simulink model "untitle2d"  (R2022a)
settings: Solver=FixedStepAuto  StartTime=0.0  StopTime=50  FixedStep=0.1  RelTol=1e-3
undefined symbols (not defined in the file): c1, k1, m1
settings Model: Creator=sucho  LastModifiedBy=sucho

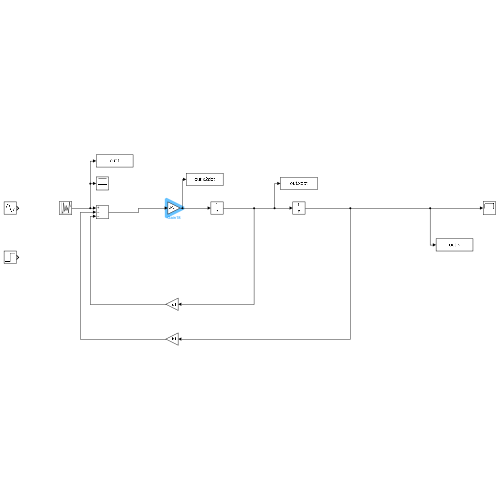
[thumbnail: Simulink's stored preview of the top-level diagram]
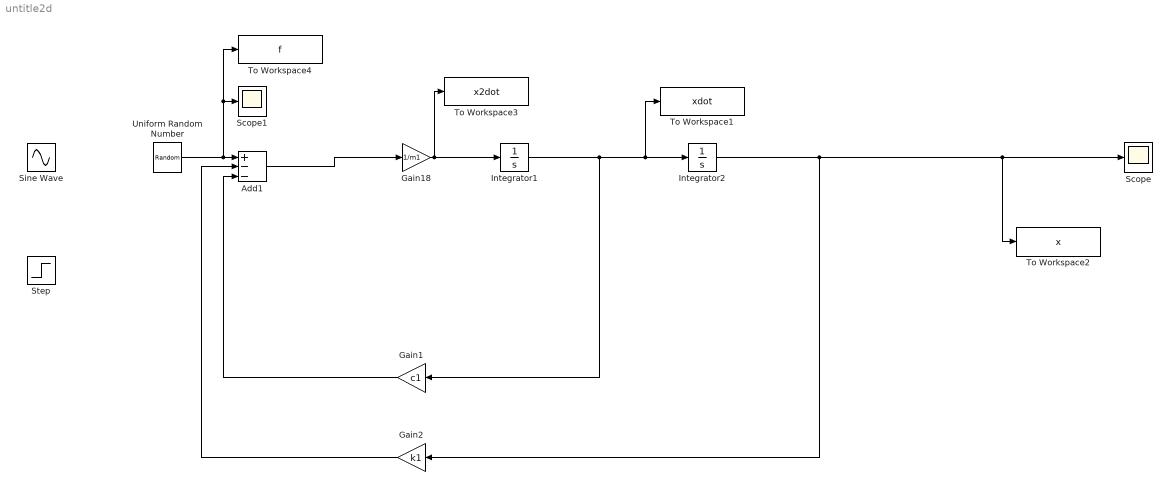
== system untitle2d ==
  Add1 : Sum  Inputs=+--
  Gain1 : Gain  Gain=c1
  Gain18 : Gain  Gain=1/m1
  Gain2 : Gain  Gain=k1
  Integrator1 : Integrator  InitialCondition=1
  Integrator2 : Integrator  InitialCondition=1
  Scope : Scope
  Scope1 : Scope
  Sine Wave : Sin  SampleTime=0
  Step : Step  SampleTime=0
  To Workspace1 : ToWorkspace  VariableName=xdot  SampleTime=0.1
  To Workspace2 : ToWorkspace  VariableName=x  SampleTime=0.1
  To Workspace3 : ToWorkspace  VariableName=x2dot  SampleTime=0.1
  To Workspace4 : ToWorkspace  VariableName=f  SampleTime=0.1
  Uniform Random Number : UniformRandomNumber  SampleTime=0.1
  wires:
  Gain1/1 -> Add1/3
  Integrator2/1 -> Scope/1, To Workspace2/1, Gain2/1
  Gain2/1 -> Add1/2
  Integrator1/1 -> Gain1/1, To Workspace1/1, Integrator2/1
  Gain18/1 -> To Workspace3/1, Integrator1/1
  Add1/1 -> Gain18/1
  Uniform Random Number/1 -> To Workspace4/1, Scope1/1, Add1/1
